simulink model "FinalPlan"  (R2019b)
settings: Solver=VariableStepAuto  StartTime=0.0  StopTime=16  RelTol=1e-3
values from neighbouring files (symbols this model uses):
  X = 1    [initialSim.m]
  Y = 1    [initialSim.m]
undefined symbols (not defined in the file or in its folder): PhiDesire, PhoDesire
libraries: simulink x3
settings Model: Creator=yuhaiyang  LastModifiedBy=yuhaiyang

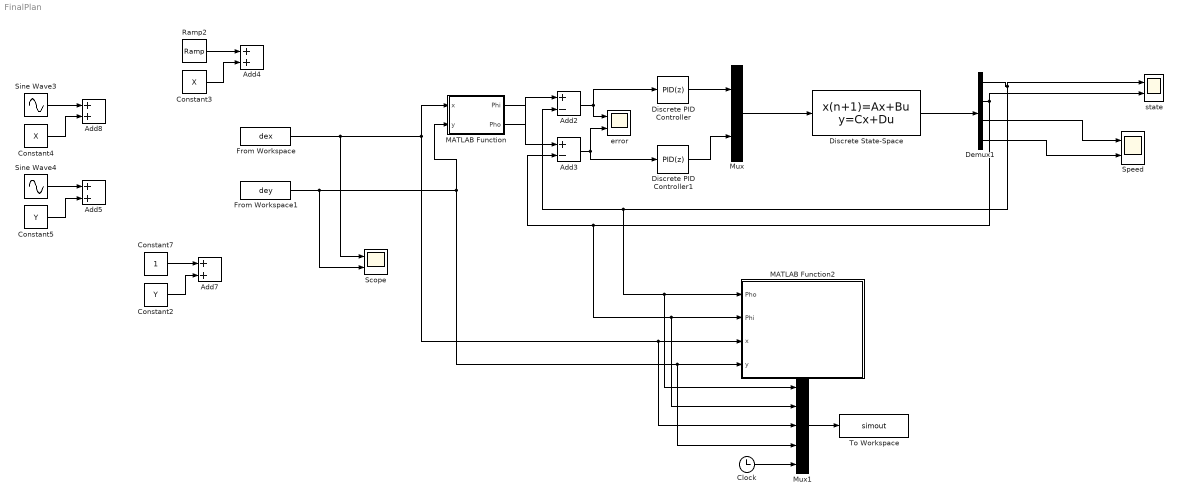
== system FinalPlan ==
  Add2 : Sum  Inputs=+-
  Add3 : Sum  Inputs=+-
  Add{4..5,7..8} (4 alike) : Sum
  Clock : Clock
  Constant2 : Constant  Value=Y
  Constant3 : Constant  Value=X
  Constant4 : Constant  Value=X
  Constant5 : Constant  Value=Y
  Constant7 : Constant
  Demux1 : Demux
  Discrete PID Controller : simulink/Continuous/PID Controller  Controller=PID  Form=Parallel  TimeDomain=Discrete-time  SampleTime=step  IntegratorMethod=Forward Euler  FilterMethod=Forward Euler  ControllerParametersSource=internal  P=0.0451594253248729  I=0.00606949033779435  D=0.0825217736897104  UseFilter=on  N=17.4747024685303  TunerSelectOption=Transfer Function Based (PID Tuner App)  InitialConditionSource=internal  InitialConditionForIntegrator=0  InitialConditionForFilter=0  DifferentiatorICPrevScaledInput=0  ExternalReset=none  TrackingMode=off  Kt=1  LimitOutput=off  UpperSaturationLimit=inf  LowerSaturationLimit=-inf  LinearizeAsGain=off  AntiWindupMode=none  Kb=1  POutMin=[]  POutMax=[]  IOutMin=[]  IOutMax=[]  DOutMin=[]  DOutMax=[]  NOutMin=[]  NOutMax=[]  SumOutMin=[]  SumOutMax=[]  SaturationOutMin=[]  SaturationOutMax=[]  PParamMin=[]  PParamMax=[]  IParamMin=[]  IParamMax=[]  DParamMin=[]  DParamMax=[]  NParamMin=[]  NParamMax=[]  KbParamMin=[]  KbParamMax=[]  KtParamMin=[]  KtParamMax=[]  KbOutMin=[]  KbOutMax=[]  KtOutMin=[]  KtOutMax=[]  IntegratorOutMin=[]  IntegratorOutMax=[]  FilterOutMin=[]  FilterOutMax=[]  SumI1OutMin=[]  SumI1OutMax=[]  SumI2OutMin=[]  SumI2OutMax=[]  SumI3OutMin=[]  SumI3OutMax=[]  SumI4OutMin=[]  SumI4OutMax=[]  SumDOutMin=[]  SumDOutMax=[]  DifferentiatorOutMin=[]  DifferentiatorOutMax=[]  FilterDiffOutCoefMin=[]  FilterDiffOutCoefMax=[]  ReciprocalOutMin=[]  ReciprocalOutMax=[]  SumDenOutMin=[]  SumDenOutMax=[]  SumNumOutMin=[]  SumNumOutMax=[]  DivideOutMin=[]  DivideOutMax=[]  IntegratorContinuousStateAttributes=''  IntegratorStateMustResolveToSignalObject=off  IntegratorRTWStateStorageClass=Auto  FilterContinuousStateAttributes=''  FilterStateMustResolveToSignalObject=off  FilterRTWStateStorageClass=Auto  ParallelPVariant=InternalParameters  IdealPVariant=Disabled  IVariant=InternalParameters  DVariant=InternalParameters  IntegratorVariant=Discrete  SatVariant=Disabled  AWVariant=Passthrough  PCopyVariant=Disabled  TRVariant=Disabled  FdbkBlocksVariant=Forward  IdealPFdbkVariant=Disabled  SatFdbkVariant=Disabled  DerivativeFilterVariant=ForwardEulerFilter  NVariant=InternalParameters  NCopyVariant=Disabled  FilterICVariant=InternalICsFilter  IntegratorICVariant=InternalICs  ExternalResetVariant=Disabled  TRSumVariant=Passthrough  SumFdbkVariant=Disabled  SumVariant=Sum_PID
  Discrete PID Controller1 : simulink/Continuous/PID Controller  Controller=PID  Form=Parallel  TimeDomain=Discrete-time  SampleTime=step  IntegratorMethod=Forward Euler  FilterMethod=Forward Euler  ControllerParametersSource=internal  P=0.0143220434066502  I=0.00109223482739123  D=0.0463013739503765  UseFilter=on  N=12.1025626011462  TunerSelectOption=Transfer Function Based (PID Tuner App)  InitialConditionSource=internal  InitialConditionForIntegrator=0  InitialConditionForFilter=0  DifferentiatorICPrevScaledInput=0  ExternalReset=none  TrackingMode=off  Kt=1  LimitOutput=off  UpperSaturationLimit=inf  LowerSaturationLimit=-inf  LinearizeAsGain=off  AntiWindupMode=none  Kb=1  POutMin=[]  POutMax=[]  IOutMin=[]  IOutMax=[]  DOutMin=[]  DOutMax=[]  NOutMin=[]  NOutMax=[]  SumOutMin=[]  SumOutMax=[]  SaturationOutMin=[]  SaturationOutMax=[]  PParamMin=[]  PParamMax=[]  IParamMin=[]  IParamMax=[]  DParamMin=[]  DParamMax=[]  NParamMin=[]  NParamMax=[]  KbParamMin=[]  KbParamMax=[]  KtParamMin=[]  KtParamMax=[]  KbOutMin=[]  KbOutMax=[]  KtOutMin=[]  KtOutMax=[]  IntegratorOutMin=[]  IntegratorOutMax=[]  FilterOutMin=[]  FilterOutMax=[]  SumI1OutMin=[]  SumI1OutMax=[]  SumI2OutMin=[]  SumI2OutMax=[]  SumI3OutMin=[]  SumI3OutMax=[]  SumI4OutMin=[]  SumI4OutMax=[]  SumDOutMin=[]  SumDOutMax=[]  DifferentiatorOutMin=[]  DifferentiatorOutMax=[]  FilterDiffOutCoefMin=[]  FilterDiffOutCoefMax=[]  ReciprocalOutMin=[]  ReciprocalOutMax=[]  SumDenOutMin=[]  SumDenOutMax=[]  SumNumOutMin=[]  SumNumOutMax=[]  DivideOutMin=[]  DivideOutMax=[]  IntegratorContinuousStateAttributes=''  IntegratorStateMustResolveToSignalObject=off  IntegratorRTWStateStorageClass=Auto  FilterContinuousStateAttributes=''  FilterStateMustResolveToSignalObject=off  FilterRTWStateStorageClass=Auto  ParallelPVariant=InternalParameters  IdealPVariant=Disabled  IVariant=InternalParameters  DVariant=InternalParameters  IntegratorVariant=Discrete  SatVariant=Disabled  AWVariant=Passthrough  PCopyVariant=Disabled  TRVariant=Disabled  FdbkBlocksVariant=Forward  IdealPFdbkVariant=Disabled  SatFdbkVariant=Disabled  DerivativeFilterVariant=ForwardEulerFilter  NVariant=InternalParameters  NCopyVariant=Disabled  FilterICVariant=InternalICsFilter  IntegratorICVariant=InternalICs  ExternalResetVariant=Disabled  TRSumVariant=Passthrough  SumFdbkVariant=Disabled  SumVariant=Sum_PID
  Discrete State-Space : DiscreteStateSpace  A=|  B=|  C=[1,0,0,0;0,1,0,0;0,0,1,0;0,0,0,1]  D=[0,0;0,0;0,0;0,0]  InitialCondition=[PhoDesire,PhiDesire,0,0]'  SampleTime=step
      A=|
      | [1,0,step,0;
      |     0,1,0,step;
      |     0,0,1,0;
      |     0,0,0,1];
      B=|
      | [0,0;
      |     0,0;
      |     100*pi/180,0;
      |     0,100*pi/180];
  From Workspace : FromWorkspace  VariableName=dex  SampleTime=0
  From Workspace1 : FromWorkspace  VariableName=dey  SampleTime=0
  MATLAB Function : MATLAB Function  TreatAsAtomicUnit=on
  MATLAB Function2 : MATLAB Function  TreatAsAtomicUnit=on
  Mux : Mux  Inputs=2
  Mux1 : Mux  Inputs=5
  Ramp2 : simulink/Sources/Ramp  slope=0.2  start=0  InitialOutput=0
  Scope : Scope  NumInputPorts=2
  Sine Wave3 : Sin  Frequency=0.5  SampleTime=step
  Sine Wave4 : Sin  Frequency=0.5  Phase=pi/2  SampleTime=step
  Speed : Scope  NumInputPorts=2
  To Workspace : ToWorkspace  VariableName=simout  SampleTime=-1
      settings: Save2DSignal=2-D array (concatenate along first dimension)
  "error " : Scope  NumInputPorts=2
  state : Scope  NumInputPorts=2
  wires:
  Ramp2/1 -> Add4/1
  Constant3/1 -> Add4/2
  Mux1/1 -> To Workspace/1
  Demux1/2 -> Mux1/2, MATLAB Function2/2(Phi), Add3/2, state/2
  Discrete PID Controller/1 -> Mux/1
  Mux/1 -> Discrete State-Space/1
  Demux1/1 -> state/1, Add2/2, Mux1/1, MATLAB Function2/1(Pho)
  MATLAB Function/1(Phi) -> Add3/1
  Discrete State-Space/1 -> Demux1/1
  Add2/1 -> Discrete PID Controller/1, "error "/1
  Discrete PID Controller1/1 -> Mux/2
  Clock/1 -> Mux1/5
  Constant2/1 -> Add7/2
  Demux1/4 -> Speed/2
  Add3/1 -> "error "/2, Discrete PID Controller1/1
  From Workspace1/1 -> Scope/2, MATLAB Function/2(y), Mux1/4, MATLAB Function2/4(y)
  MATLAB Function/2(Pho) -> Add2/1
  Demux1/3 -> Speed/1
  Constant7/1 -> Add7/1
  Sine Wave3/1 -> Add8/1
  Constant5/1 -> Add5/2
  From Workspace/1 -> Scope/1, MATLAB Function/1(x), Mux1/3, MATLAB Function2/3(x)
  Sine Wave4/1 -> Add5/1
  Constant4/1 -> Add8/2

== matlab function FinalPlan/MATLAB Function ==
  data: x input; Phi output; y input; Pho output
function [Phi,Pho] = fcn(x,y)
z = 0;
X = 1;
Y = 1;
Z = 6;

dist = sqrt((x-X)^2+(y-Y)^2+(z-Z)^2);
Phi = acos((z-Z)/dist);

if y<Y
    Pho = atan(-(x-X)/(y-Y));
elseif y>Y
    Pho = pi+atan(-(x-X)/(y-Y));
else
    if x>X
        Pho = pi/2;
    else
        Pho = pi+pi/2;
    end
end

== matlab function FinalPlan/MATLAB Function2 ==
  data: Pho input; Phi input; x input; y input
function detectPlot2(Pho,Phi,x,y)

X = 1;
Y = 1;
Z = 6;
z = 0;
axis([-1 3.5 -1 3.5,0,6])
detect2(X,Y,Z,Pho,Phi);
alpha(0.25);
hold on
%plot3(x,y,z,'r*')
hold off
axis([-1 3.5 -1 3.5,0,6])
